simulink model "meam_simulink"  (R2020a)
settings: Solver=FixedStepAuto  StartTime=0.0  StopTime=10.0  FixedStep=0.0001  RelTol=1e-3
undefined symbols (not defined in the file): cnc_comp, ctc_switch, ctrl_at_end, ctrl_space, delta, ea_set_1, ea_set_2, ee_att_1, ee_att_2, f_des, force_ffwd, fp_1, fp_2, frc_comp, grv_comp, ip_1, ip_2, K, Kc, Kd, Kdf, Ki, Kif, Km, Kp, Kpf, orn_at_norm, prdc_frc, q_posIni, q_posIni_1, robot_model_1, robot_model_2, rpt_num_1, rpt_num_2, Sf_diag, spr_comp, switch_val, Sx_diag, tf_1, tf_2, trj_at_end, trj_profile_1, trj_profile_2, trj_space_1, trj_space_2, trj_type_1, trj_type_2
libraries: simulink x2, vrlib x1
(part 1 of 4)
settings Model: Creator=Mertcan  LastModifiedBy=Mertcan

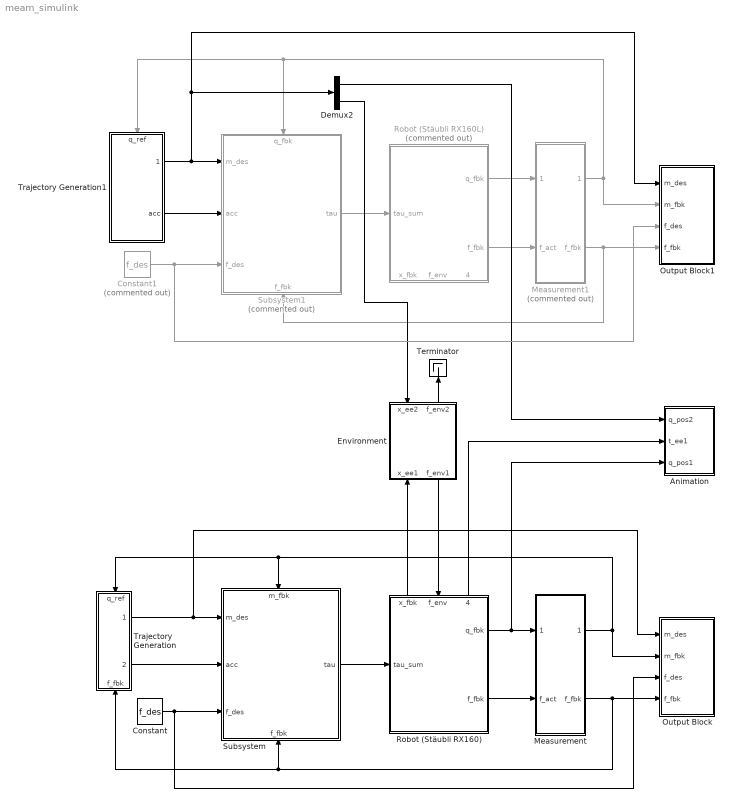
== system meam_simulink ==
  Animation : Subsystem
  Constant : Constant  Value=f_des
  Constant1 : Constant  Commented=on  Value=f_des
  Demux2 : Demux  Outputs=[12;18]
  Environment : Subsystem
      settings: PortSchema="{\"entries\":[{\"content\":{\"sides\":[{\"content\":{\"connectorIds\":[]},\"type\":\"ConnectorPlacement.EquallySpacedRectSide\",\"uuid\":\"b81f9d7c-ea51-4f8c-a6d1-c33009541a36\"},{\"content\":{\"connectorIds\":[],\"side\":\"RIGHT\"},\"type\":\"ConnectorPlacement.EquallySpacedRectSide\",\"uuid\":\"c20f2b2d-2c64-4ed8-b53c-24ad73d5cd54\"},{\"content\":{\"connectorIds\":[\"In1\",\"Out2\"],\"side\":\"TOP\"},\"type\":\"ConnectorPlacement.EquallySpacedRectSide\",\"uuid\":\"f43a164f-97c5-4b00-9b12-265fb19428de\"},{\"content\":{\"connectorIds\":[\"In2\",\"Out1\"],\"side\":\"BOTTOM\"},\"type\":\"ConnectorPlacement.EquallySpacedRectSide\",\"uuid\":\"d7f17a50-52f4-4125-8d61-9ac09671e8dc\"}]},\"type\":\"ConnectorPlacement.EquallySpacedConnector\",\"uuid\":\"950c3a05-8add-442a-8ea6-c018fdaf9f56\"}],\"packageUris\":[\"http://schema.mathworks.com/mf0/Connector/19700101\"],\"version\":\"1.0\"}"
  Measurement : Subsystem
  Measurement1 : Subsystem  Commented=on
  Output Block : Subsystem
  Output Block1 : Subsystem
  Robot (Stäubli RX160) : Subsystem
      settings: PortSchema="{\"entries\":[{\"content\":{\"sides\":[{\"content\":{\"connectorIds\":[\"In1\"]},\"type\":\"ConnectorPlacement.EquallySpacedRectSide\",\"uuid\":\"6284adc3-d758-45ef-9141-dee680c83b08\"},{\"content\":{\"connectorIds\":[\"Out1\",\"Out2\"],\"side\":\"RIGHT\"},\"type\":\"ConnectorPlacement.EquallySpacedRectSide\",\"uuid\":\"181d7ec4-49ad-445a-9254-c2b56cfcaf16\"},{\"content\":{\"connectorIds\":[\"Out3\",\"In2\",\"Out4\"],\"side\":\"TOP\"},\"type\":\"ConnectorPlacement.EquallySpacedRectSide\",\"uuid\":\"b714267f-2932-4320-9de1-3f424c8ad2a6\"}]},\"type\":\"ConnectorPlacement.EquallySpacedConnector\",\"uuid\":\"69d7b4c6-737c-4cfe-af82-254ae10a5bd4\"}],\"packageUris\":[\"http://schema.mathworks.com/mf0/Connector/19700101\"],\"version\":\"1.0\"}"
      mask Display: image('$imagefile'); % Use "Edit Image" on toolstrip to change.
  Robot (Stäubli RX160L) : Subsystem  Commented=on
      settings: PortSchema="{\"entries\":[{\"content\":{\"sides\":[{\"content\":{\"connectorIds\":[\"In1\"]},\"type\":\"ConnectorPlacement.EquallySpacedRectSide\",\"uuid\":\"6284adc3-d758-45ef-9141-dee680c83b08\"},{\"content\":{\"connectorIds\":[\"Out1\",\"Out2\"],\"side\":\"RIGHT\"},\"type\":\"ConnectorPlacement.EquallySpacedRectSide\",\"uuid\":\"181d7ec4-49ad-445a-9254-c2b56cfcaf16\"},{\"content\":{\"connectorIds\":[],\"side\":\"TOP\"},\"type\":\"ConnectorPlacement.EquallySpacedRectSide\",\"uuid\":\"b714267f-2932-4320-9de1-3f424c8ad2a6\"},{\"content\":{\"connectorIds\":[\"Out3\",\"In2\",\"Out4\"],\"side\":\"BOTTOM\"},\"type\":\"ConnectorPlacement.EquallySpacedRectSide\",\"uuid\":\"b9e977bd-f5b6-4bc7-a651-d9aa29860466\"}]},\"type\":\"ConnectorPlacement.EquallySpacedConnector\",\"uuid\":\"69d7b4c6-737c-4cfe-af82-254ae10a5bd4\"}],\"packageUris\":[\"http://schema.mathworks.com/mf0/Connector/19700101\"],\"version\":\"1.0\"}"
      mask Display: image('$imagefile'); % Use "Edit Image" on toolstrip to change.
  Subsystem : Subsystem
      settings: PortSchema="{\"entries\":[{\"content\":{\"sides\":[{\"content\":{\"connectorIds\":[\"In1\",\"In2\",\"In3\"]},\"type\":\"ConnectorPlacement.EquallySpacedRectSide\",\"uuid\":\"06a54d02-8053-40c1-91cd-d8e27b3ee47c\"},{\"content\":{\"connectorIds\":[\"Out1\"],\"side\":\"RIGHT\"},\"type\":\"ConnectorPlacement.EquallySpacedRectSide\",\"uuid\":\"4a80d155-eaa4-4553-b775-68e65830b71e\"},{\"content\":{\"connectorIds\":[\"In4\"],\"side\":\"TOP\"},\"type\":\"ConnectorPlacement.EquallySpacedRectSide\",\"uuid\":\"11a6b61a-4e29-4238-936c-c215c9d368a9\"},{\"content\":{\"connectorIds\":[\"In5\"],\"side\":\"BOTTOM\"},\"type\":\"ConnectorPlacement.EquallySpacedRectSide\",\"uuid\":\"e426367f-91c4-44b7-ba01-8266a65ceab9\"}]},\"type\":\"ConnectorPlacement.EquallySpacedConnector\",\"uuid\":\"b69ba746-893b-40a9-a2ce-44750d5af8bd\"}],\"packageUris\":[\"http://schema.mathworks.com/mf0/Connector/19700101\"],\"version\":\"1.0\"}"
  Subsystem1 : Subsystem  Commented=on
      settings: PortSchema="{\"entries\":[{\"content\":{\"sides\":[{\"content\":{\"connectorIds\":[\"In1\",\"In2\",\"In3\"]},\"type\":\"ConnectorPlacement.EquallySpacedRectSide\",\"uuid\":\"cd98d980-3223-4404-96a3-1b871aee0cda\"},{\"content\":{\"connectorIds\":[\"Out1\"],\"side\":\"RIGHT\"},\"type\":\"ConnectorPlacement.EquallySpacedRectSide\",\"uuid\":\"917be7da-8185-449c-972b-8d7b61571565\"},{\"content\":{\"connectorIds\":[\"In4\"],\"side\":\"TOP\"},\"type\":\"ConnectorPlacement.EquallySpacedRectSide\",\"uuid\":\"910fa89e-4196-4c93-9d4c-b419700893fa\"},{\"content\":{\"connectorIds\":[\"In5\"],\"side\":\"BOTTOM\"},\"type\":\"ConnectorPlacement.EquallySpacedRectSide\",\"uuid\":\"8581f1c3-c928-4a87-9392-429d43b2dbef\"}]},\"type\":\"ConnectorPlacement.EquallySpacedConnector\",\"uuid\":\"8ec3d0f0-5e55-41fc-8255-3218c3c2560b\"}],\"packageUris\":[\"http://schema.mathworks.com/mf0/Connector/19700101\"],\"version\":\"1.0\"}"
  Terminator : Terminator
  Trajectory Generation : Subsystem
      settings: PortSchema="{\"entries\":[{\"content\":{\"sides\":[{\"content\":{\"connectorIds\":[]},\"type\":\"ConnectorPlacement.EquallySpacedRectSide\",\"uuid\":\"88b86860-d81b-4a43-9b48-bb84105d3d48\"},{\"content\":{\"connectorIds\":[\"Out1\",\"Out2\"],\"side\":\"RIGHT\"},\"type\":\"ConnectorPlacement.EquallySpacedRectSide\",\"uuid\":\"c294309b-61d9-4e8b-865e-5d40c6635825\"},{\"content\":{\"connectorIds\":[\"In1\"],\"side\":\"TOP\"},\"type\":\"ConnectorPlacement.EquallySpacedRectSide\",\"uuid\":\"9b2aaf3f-7cff-4a7a-8968-0748d2e865cd\"},{\"content\":{\"connectorIds\":[\"In2\"],\"side\":\"BOTTOM\"},\"type\":\"ConnectorPlacement.EquallySpacedRectSide\",\"uuid\":\"3b326038-a616-4ec6-89ef-aa45e9a74c57\"}]},\"type\":\"ConnectorPlacement.EquallySpacedConnector\",\"uuid\":\"563f6bfd-f175-4769-9892-8fc54dd6cf01\"}],\"packageUris\":[\"http://schema.mathworks.com/mf0/Connector/19700101\"],\"version\":\"1.0\"}"
  Trajectory Generation1 : Subsystem
      settings: PortSchema="{\"entries\":[{\"content\":{\"sides\":[{\"content\":{\"connectorIds\":[]},\"type\":\"ConnectorPlacement.EquallySpacedRectSide\",\"uuid\":\"4512f7c1-141f-4ca9-8985-d7b3fc7dc203\"},{\"content\":{\"connectorIds\":[\"Out1\",\"Out2\"],\"side\":\"RIGHT\"},\"type\":\"ConnectorPlacement.EquallySpacedRectSide\",\"uuid\":\"5c5a9662-9ae9-4eb5-828e-be3fe6f4b168\"},{\"content\":{\"connectorIds\":[\"In1\"],\"side\":\"TOP\"},\"type\":\"ConnectorPlacement.EquallySpacedRectSide\",\"uuid\":\"4c26be9f-0fe4-4a1d-a76a-786ec65b737d\"},{\"content\":{\"connectorIds\":[],\"side\":\"BOTTOM\"},\"type\":\"ConnectorPlacement.EquallySpacedRectSide\",\"uuid\":\"9d756de9-72bc-4633-ac1d-40b2671d614a\"}]},\"type\":\"ConnectorPlacement.EquallySpacedConnector\",\"uuid\":\"303d3c57-cadd-4518-8f0b-ca4d9a4186ef\"}],\"packageUris\":[\"http://schema.mathworks.com/mf0/Connector/19700101\"],\"version\":\"1.0\"}"
  wires:
  Constant/1 -> Subsystem/3(f_des), Output Block/3(f_des)
  Measurement1/1(m_fbk) -> Output Block1/2(m_fbk), Trajectory Generation1/1(q_ref), Subsystem1/4(q_fbk)
  Environment/2(f_env2) -> Terminator/1
  Trajectory Generation1/1(pos&vel) -> Output Block1/1(m_des), Demux2/1, Subsystem1/1(m_des)
  Trajectory Generation/1(pos&vel) -> Output Block/1(m_des), Subsystem/1(m_des)
  Subsystem1/1(tau) -> Robot (Stäubli RX160L)/1(tau_sum)
  Robot (Stäubli RX160L)/1(q_fbk) -> Measurement1/1(q_act)
  Measurement/1(m_fbk) -> Output Block/2(m_fbk), Trajectory Generation/1(q_ref), Subsystem/4(m_fbk)
  Measurement1/2(f_fbk) -> Subsystem1/5(f_fbk), Output Block1/4(f_fbk)
  Robot (Stäubli RX160L)/2(f_fbk) -> Measurement1/2(f_act)
  Demux2/1 -> Animation/1(q_pos2)
  Subsystem/1(tau) -> Robot (Stäubli RX160)/1(tau_sum)
  Demux2/2 -> Environment/1(x_ee2)
  Environment/1(f_env1) -> Robot (Stäubli RX160)/2(f_env)
  Trajectory Generation/2(acc) -> Subsystem/2(acc)
  Robot (Stäubli RX160)/2(f_fbk) -> Measurement/2(f_act)
  Constant1/1 -> Output Block1/3(f_des), Subsystem1/3(f_des)
  Robot (Stäubli RX160)/4(x_compress) -> Animation/2(t_ee1)
  Measurement/2(f_fbk) -> Output Block/4(f_fbk), Trajectory Generation/2(f_fbk), Subsystem/5(f_fbk)
  Robot (Stäubli RX160)/1(q_fbk) -> Measurement/1(q_act), Animation/3(q_pos1)
  Robot (Stäubli RX160)/3(x_fbk) -> Environment/2(x_ee1)
  Trajectory Generation1/2(acc) -> Subsystem1/2(acc)

== system meam_simulink/Animation ==
  q_pos2 : Inport
  t_ee1 : Inport  Port=2
  q_pos1 : Inport  Port=3
  Constant : Constant  Value=1e3
  Demux : Demux  Outputs=2
  Demux1 : Demux  Outputs=2
  Demux2 : Demux  Outputs=3
  Product : Product
  Terminator{,1..3} (4 alike) : Terminator
  To Workspace1 : ToWorkspace  VariableName=eePosCompress  SaveFormat=Timeseries  SampleTime=-1
  VR Sink1 : vrlib/VR Sink  InstantiateOnLoad=on  SampleTime=0.1  ViewEnable=on  RemoteChange=off  RemoteView=off  FieldsWritten=joint_joint_1.rotation.4.1.1.double#joint_joint_2.rotation.4.1.1.double#joint_joint_3.rotation.4.1.1.double#joint_joint_4.rotation.4.1.1.double#joint_joint_5.rotation.4.1.1.double#joint_joint_6.rotation.4.1.1.double#rod_sphere.translation.3.1.1.double#joint_joint_1_0001.rotation.4.1.1.double#joint_joint_2_0001.rotation.4.1.1.double#joint_joint_3_0001.rotation.4.1.1.double#joint_joint_4_0001.rotation.4.1.1.double#joint_joint_5_0001.rotation.4.1.1.double#joint_joint_6_0001.rotation.4.1.1.double  WorldFileName=vr_two_robots_base.x3d  WorldDescription=Dual Robot Scene  AutoView=on  VideoDimensions=[]  AllowVariableSize=off  FigureProperties="{'Position', 'Name', 'Viewpoint', 'CameraBound', 'CameraDirection', 'CameraPosition', 'CameraUpVector', 'ZoomFactor', 'Antialiasing', 'Headlight', 'Lighting', 'NavPanel', 'Sound', 'StatusBar', 'Stereo3D', 'Stereo3DCameraOffset', 'Stereo3DHIT', 'ToolBar', 'Textures', 'Transparency', 'Triad', 'Wireframe', 'NavZones', 'NavMode', 'NavSpeed', 'CaptureFileFormat', 'CaptureFileName', 'Record2DCompressMethod', 'Record2DCompressQuality', 'Record2D', 'Record2DFileName', 'Record2DFPS'; [7.0100000000000000e+02   2.6000000000000000e+02   1.1860000000000000e+03   6.6700000000000000e+02], 'Dual Robot Scene', 'Close View', 'on', [9.6576292467919089e-01  -1.3282628958850401e-01   2.2284333086116798e-01], [-4.0999222072425230e+00   7.2376690346139994e-01  -4.0692759072460811e+00], [1.1281783288456564e-01   9.8854135680228927e-01   1.0029019131923340e-01], [1.0000000000000000e+00], 'on', 'on', 'on', 'halfbar', 'on', 'on', 'off', [1.0000000149011612e-01], [0.0000000000000000e+00], 'on', 'on', 'on', 'none', 'off', 'off', 'examine', 'normal', 'tif', '%f_anim_%n.tif', 'auto', [7.5000000000000000e+01], 'off', '%f_anim_%n.avi', 'auto'}"
  Zero-Order Hold : ZeroOrderHold  SampleTime=0.004
  fwd kin : MATLAB Function  TreatAsAtomicUnit=on
  fwd kin1 : MATLAB Function  TreatAsAtomicUnit=on
  wires:
  q_pos1/1 -> Demux/1
  Demux/1 -> fwd kin/1(u)
  Demux/2 -> Terminator/1
  q_pos2/1 -> Demux1/1
  Demux1/2 -> Terminator1/1
  Demux1/1 -> fwd kin1/1(u)
  fwd kin/1(r1) -> VR Sink1/1
  fwd kin/2(r2) -> VR Sink1/2
  fwd kin/3(r3) -> VR Sink1/3
  fwd kin/4(r4) -> VR Sink1/4
  fwd kin/5(r5) -> VR Sink1/5
  fwd kin/6(r6) -> VR Sink1/6
  fwd kin1/1(r1) -> VR Sink1/8
  fwd kin1/2(r2) -> VR Sink1/9
  fwd kin1/3(r3) -> VR Sink1/10
  fwd kin1/4(r4) -> VR Sink1/11
  fwd kin1/5(r5) -> VR Sink1/12
  fwd kin1/6(r6) -> VR Sink1/13
  t_ee1/1 -> Product/2, Demux2/1
  Product/1 -> VR Sink1/7
  Constant/1 -> Product/1
  Demux2/1 -> Terminator2/1
  Demux2/2 -> Terminator3/1
  Zero-Order Hold/1 -> To Workspace1/1
  Demux2/3 -> Zero-Order Hold/1

== system meam_simulink/Environment ==
  x_ee2 : Inport
  x_ee1 : Inport  Port=2
  Clock : Clock  Commented=on
  Constant : Constant  Value=-1
  Constant2 : Constant  Commented=on  Value=[0;0;0]
  MATLAB Function : MATLAB Function  Commented=on  TreatAsAtomicUnit=on
  MATLAB Function1 : MATLAB Function  TreatAsAtomicUnit=on
  MATLAB Function2 : MATLAB Function  Commented=on  TreatAsAtomicUnit=on
  MATLAB Function3 : MATLAB Function  Commented=on  TreatAsAtomicUnit=on
  Product : Product
  Scope : Scope  Commented=on
  Stifness : Constant  Commented=on  Value=K
  Stifness1 : Constant  Value=K
  To Workspace1 : ToWorkspace  Commented=on  VariableName=obsPos  SaveFormat=Timeseries  SampleTime=-1
  delta : Constant  Commented=on  Value=delta
  end-effector attach : Constant  Value=ee_att_1
  f_env1 : Outport
  f_env2 : Outport  Port=2
  wires:
  Stifness/1 -> MATLAB Function/1(K)
  Clock/1 -> MATLAB Function/4(t)
  MATLAB Function/2(x) -> To Workspace1/1, Scope/1
  delta/1 -> MATLAB Function/2(delta)
  x_ee2/1 -> MATLAB Function1/3(x2)
  Product/1 -> f_env2/1
  x_ee1/1 -> MATLAB Function1/1(x1)  "x"
  Stifness1/1 -> MATLAB Function1/4(K)
  MATLAB Function1/1(f_e) -> Product/2, f_env1/1
  Constant2/1 -> MATLAB Function/3(u)
  Constant/1 -> Product/1
  end-effector attach/1 -> MATLAB Function1/2(ee_att_1)

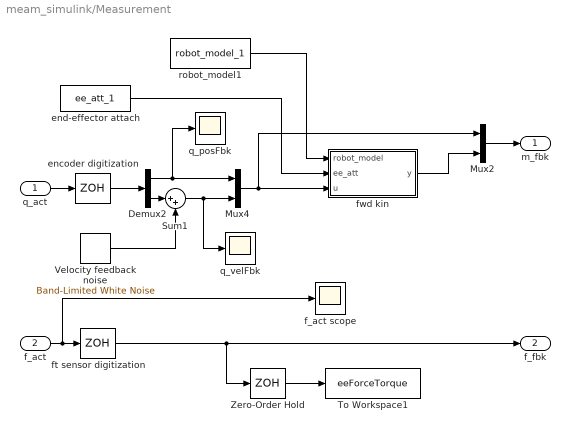
== system meam_simulink/Measurement ==
  q_act : Inport
  f_act : Inport  Port=2
  Demux2 : Demux  Outputs=2
  Mux2 : Mux  Inputs=[12;18]
  Mux4 : Mux  Inputs=2
  Sum1 : Sum  Inputs=|++
  To Workspace1 : ToWorkspace  VariableName=eeForceTorque  SaveFormat=Timeseries  SampleTime=-1
  Velocity feedback noise : simulink/Sources/Band-Limited White Noise  Cov=[0.00001]  Ts=0.01  seed=[23341]
  Zero-Order Hold : ZeroOrderHold  SampleTime=0.004
  encoder digitization : ZeroOrderHold  SampleTime=0.004
  end-effector attach : Constant  Value=ee_att_1
  f_act scope : Scope
  ft sensor digitization : ZeroOrderHold  SampleTime=0.004
  fwd kin : MATLAB Function  TreatAsAtomicUnit=on
  q_posFbk : Scope
  q_velFbk : Scope
  robot_model1 : Constant  Value=robot_model_1
  m_fbk : Outport
  f_fbk : Outport  Port=2
  wires:
  ft sensor digitization/1 -> f_fbk/1, Zero-Order Hold/1
  f_act/1 -> f_act scope/1, ft sensor digitization/1
  q_act/1 -> encoder digitization/1
  robot_model1/1 -> fwd kin/1(robot_model)
  fwd kin/1(y) -> Mux2/2
  Mux2/1 -> m_fbk/1
  Demux2/1 -> q_posFbk/1, Mux4/1
  encoder digitization/1 -> Demux2/1
  Mux4/1 -> fwd kin/3(u), Mux2/1
  Demux2/2 -> Sum1/1
  Sum1/1 -> q_velFbk/1, Mux4/2
  Velocity feedback noise/1 -> Sum1/2
  end-effector attach/1 -> fwd kin/2(ee_att)
  Zero-Order Hold/1 -> To Workspace1/1

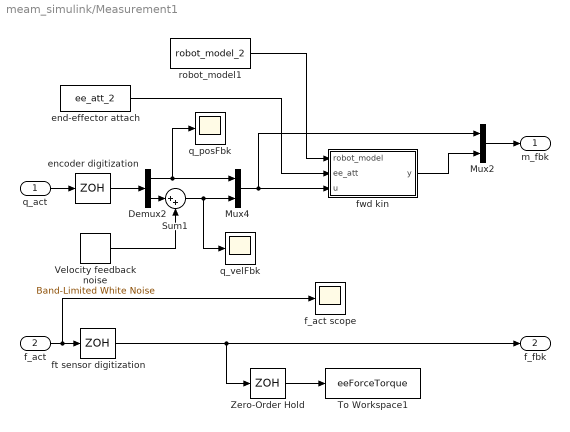
== system meam_simulink/Measurement1 ==
  q_act : Inport
  f_act : Inport  Port=2
  Demux2 : Demux  Outputs=2
  Mux2 : Mux  Inputs=[12;18]
  Mux4 : Mux  Inputs=2
  Sum1 : Sum  Inputs=|++
  To Workspace1 : ToWorkspace  VariableName=eeForceTorque  SaveFormat=Timeseries  SampleTime=-1
  Velocity feedback noise : simulink/Sources/Band-Limited White Noise  Cov=[0.00001]  Ts=0.01  seed=[23341]
  Zero-Order Hold : ZeroOrderHold  SampleTime=0.004
  encoder digitization : ZeroOrderHold  SampleTime=0.004
  end-effector attach : Constant  Value=ee_att_2
  f_act scope : Scope
  ft sensor digitization : ZeroOrderHold  SampleTime=0.004
  fwd kin : MATLAB Function  TreatAsAtomicUnit=on
  q_posFbk : Scope
  q_velFbk : Scope
  robot_model1 : Constant  Value=robot_model_2
  m_fbk : Outport
  f_fbk : Outport  Port=2
  wires:
  ft sensor digitization/1 -> f_fbk/1, Zero-Order Hold/1
  f_act/1 -> f_act scope/1, ft sensor digitization/1
  q_act/1 -> encoder digitization/1
  robot_model1/1 -> fwd kin/1(robot_model)
  fwd kin/1(y) -> Mux2/2
  Mux2/1 -> m_fbk/1
  Demux2/1 -> q_posFbk/1, Mux4/1
  encoder digitization/1 -> Demux2/1
  Mux4/1 -> fwd kin/3(u), Mux2/1
  Demux2/2 -> Sum1/1
  Sum1/1 -> q_velFbk/1, Mux4/2
  Velocity feedback noise/1 -> Sum1/2
  end-effector attach/1 -> fwd kin/2(ee_att)
  Zero-Order Hold/1 -> To Workspace1/1

== system meam_simulink/Output Block ==
  m_des : Inport
  m_fbk : Inport  Port=2
  f_des : Inport  Port=3
  f_fbk : Inport  Port=4
  Demux : Demux  Outputs=2
  Demux1 : Demux  Outputs=2
  Demux2 : Demux  Outputs=[12;18]
  Demux3 : Demux  Outputs=[12;18]
  Scope : Scope  NumInputPorts=2
  Scope1 : Scope  NumInputPorts=2
  Scope2 : Scope
  Scope3 : Scope
  Terminator{,1..3} (4 alike) : Terminator
  To Workspace : ToWorkspace  VariableName=jointPosFbk  SaveFormat=Timeseries  SampleTime=-1
  To Workspace1 : ToWorkspace  VariableName=jointPosDes  SaveFormat=Timeseries  SampleTime=-1
  wires:
  Demux/2 -> Scope1/2
  Demux1/2 -> Scope1/1
  m_des/1 -> Demux2/1
  Demux2/1 -> Demux1/1
  Demux/1 -> Scope/2, To Workspace/1
  Demux1/1 -> Scope3/1, To Workspace1/1, Scope/1
  m_fbk/1 -> Demux3/1
  Demux3/1 -> Demux/1
  Demux3/2 -> Terminator/1
  Demux2/2 -> Terminator1/1
  f_des/1 -> Terminator2/1
  f_fbk/1 -> Scope2/1, Terminator3/1

== system meam_simulink/Output Block1 ==
  m_des : Inport
  m_fbk : Inport  Port=2
  f_des : Inport  Port=3
  f_fbk : Inport  Port=4
  Demux : Demux  Commented=on  Outputs=2
  Demux1 : Demux  Outputs=2
  Demux2 : Demux  Outputs=[12;18]
  Demux3 : Demux  Commented=on  Outputs=[12;18]
  Scope : Scope  Commented=on  NumInputPorts=2
  Scope1 : Scope  Commented=on  NumInputPorts=2
  Scope2 : Scope  Commented=on
  Scope3 : Scope
  Terminator : Terminator  Commented=on
  Terminator1 : Terminator
  Terminator2 : Terminator  Commented=on
  Terminator3 : Terminator  Commented=on
  To Workspace : ToWorkspace  Commented=on  VariableName=jointPosFbk  SaveFormat=Timeseries  SampleTime=-1
  To Workspace1 : ToWorkspace  VariableName=jointPosDes2  SaveFormat=Timeseries  SampleTime=-1
  Zero-Order Hold2 : ZeroOrderHold  SampleTime=0.004
  wires:
  Demux/2 -> Scope1/2
  Demux1/2 -> Scope1/1
  m_des/1 -> Demux2/1
  Demux2/1 -> Demux1/1
  Demux/1 -> Scope/2, To Workspace/1
  Demux1/1 -> Scope3/1, Zero-Order Hold2/1, Scope/1
  m_fbk/1 -> Demux3/1
  Demux3/1 -> Demux/1
  Demux3/2 -> Terminator/1
  Demux2/2 -> Terminator1/1
  f_des/1 -> Terminator2/1
  f_fbk/1 -> Scope2/1, Terminator3/1
  Zero-Order Hold2/1 -> To Workspace1/1

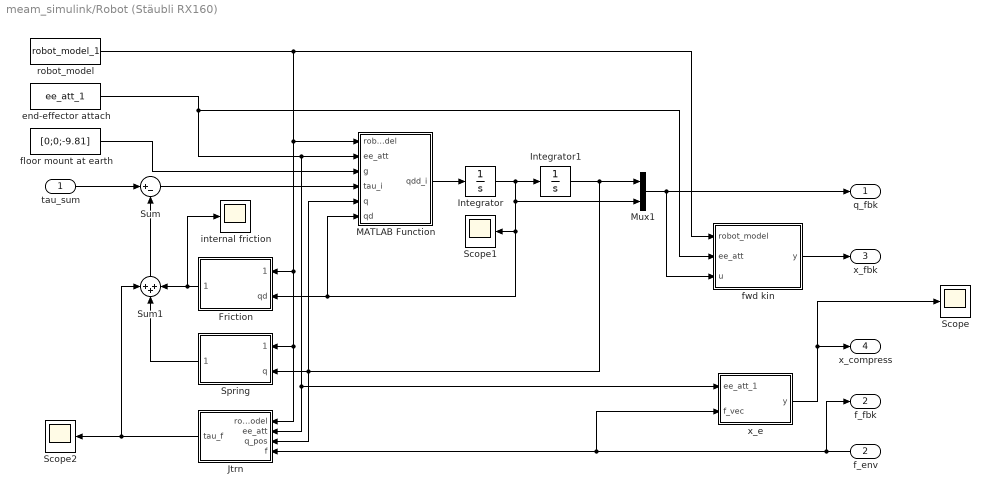
== system meam_simulink/Robot (Stäubli RX160) ==
  tau_sum : Inport
  f_env : Inport  Port=2
  Friction : MATLAB Function  TreatAsAtomicUnit=on
  Integrator : Integrator
  Integrator1 : Integrator  InitialCondition=q_posIni_1
  Jtrn : MATLAB Function  TreatAsAtomicUnit=on
  MATLAB Function : MATLAB Function  TreatAsAtomicUnit=on
  Mux1 : Mux  Inputs=2
  Scope : Scope
  Scope1 : Scope
  Scope2 : Scope
  Spring : MATLAB Function  TreatAsAtomicUnit=on
  Sum : Sum  Inputs=|+-
  Sum1 : Sum  Inputs=+++
  end-effector attach : Constant  Value=ee_att_1
  floor mount at earth : Constant  Value=[0;0;-9.81]
  fwd kin : MATLAB Function  TreatAsAtomicUnit=on
  internal friction : Scope
  robot_model : Constant  Value=robot_model_1
  x_e : MATLAB Function  TreatAsAtomicUnit=on
  q_fbk : Outport
  f_fbk : Outport  Port=2
  x_fbk : Outport  Port=3
  x_compress : Outport  Port=4
  wires:
  MATLAB Function/1(qdd_i) -> Integrator/1
  Sum/1 -> MATLAB Function/4(tau_i)
  Integrator1/1 -> Jtrn/3(q_pos), MATLAB Function/5(q), Spring/2(q), Mux1/1
  Integrator/1 -> MATLAB Function/6(qd), Friction/2(qd), Scope1/1, Mux1/2, Integrator1/1
  Friction/1(tau_frc) -> Sum1/3, internal friction/1
  Spring/1(tau_spr) -> Sum1/2
  robot_model/1 -> Jtrn/1(robot_model), Spring/1(robot_model), Friction/1(robot_model), MATLAB Function/1(robot_model), fwd kin/1(robot_model)
  Mux1/1 -> q_fbk/1, fwd kin/3(u)
  fwd kin/1(y) -> x_fbk/1
  Sum1/1 -> Sum/2
  tau_sum/1 -> Sum/1
  f_env/1 -> f_fbk/1, x_e/2(f_vec), Jtrn/4(f)
  Jtrn/1(tau_f) -> Sum1/1, Scope2/1
  end-effector attach/1 -> MATLAB Function/2(ee_att), Jtrn/2(ee_att), x_e/1(ee_att_1), fwd kin/2(ee_att)
  floor mount at earth/1 -> MATLAB Function/3(g)
  x_e/1(y) -> Scope/1, x_compress/1

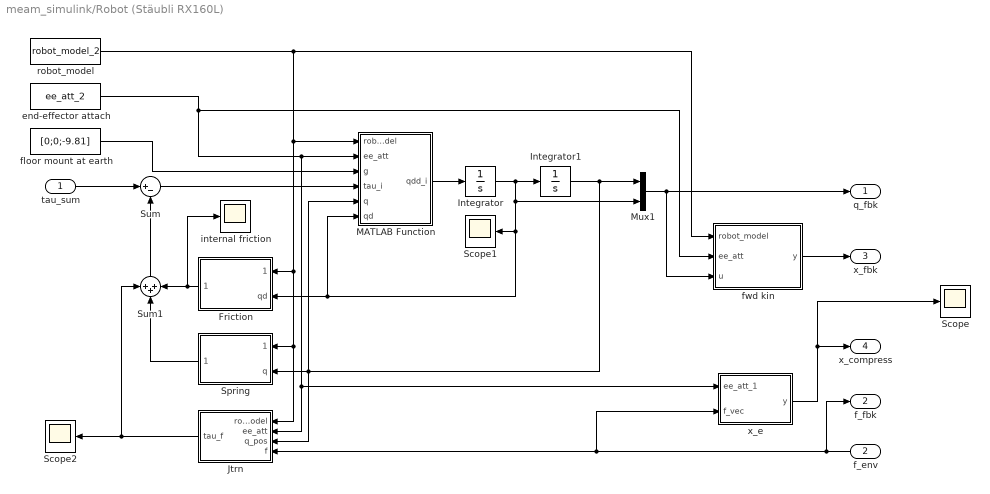
== system meam_simulink/Robot (Stäubli RX160L) ==
  tau_sum : Inport
  f_env : Inport  Port=2
  Friction : MATLAB Function  TreatAsAtomicUnit=on
  Integrator : Integrator
  Integrator1 : Integrator  InitialCondition=q_posIni
  Jtrn : MATLAB Function  TreatAsAtomicUnit=on
  MATLAB Function : MATLAB Function  TreatAsAtomicUnit=on
  Mux1 : Mux  Inputs=2
  Scope : Scope
  Scope1 : Scope
  Scope2 : Scope
  Spring : MATLAB Function  TreatAsAtomicUnit=on
  Sum : Sum  Inputs=|+-
  Sum1 : Sum  Inputs=+++
  end-effector attach : Constant  Value=ee_att_2
  floor mount at earth : Constant  Value=[0;0;-9.81]
  fwd kin : MATLAB Function  TreatAsAtomicUnit=on
  internal friction : Scope
  robot_model : Constant  Value=robot_model_2
  x_e : MATLAB Function  TreatAsAtomicUnit=on
  q_fbk : Outport
  f_fbk : Outport  Port=2
  x_fbk : Outport  Port=3
  x_compress : Outport  Port=4
  wires:
  MATLAB Function/1(qdd_i) -> Integrator/1
  Sum/1 -> MATLAB Function/4(tau_i)
  Integrator1/1 -> Jtrn/3(q_pos), MATLAB Function/5(q), Spring/2(q), Mux1/1
  Integrator/1 -> MATLAB Function/6(qd), Friction/2(qd), Scope1/1, Mux1/2, Integrator1/1
  Friction/1(tau_frc) -> Sum1/3, internal friction/1
  Spring/1(tau_spr) -> Sum1/2
  robot_model/1 -> Jtrn/1(robot_model), Spring/1(robot_model), Friction/1(robot_model), MATLAB Function/1(robot_model), fwd kin/1(robot_model)
  Mux1/1 -> q_fbk/1, fwd kin/3(u)
  fwd kin/1(y) -> x_fbk/1
  Sum1/1 -> Sum/2
  tau_sum/1 -> Sum/1
  f_env/1 -> f_fbk/1, x_e/2(f_vec), Jtrn/4(f)
  Jtrn/1(tau_f) -> Sum1/1, Scope2/1
  end-effector attach/1 -> MATLAB Function/2(ee_att), Jtrn/2(ee_att), x_e/1(ee_att_1), fwd kin/2(ee_att)
  floor mount at earth/1 -> MATLAB Function/3(g)
  x_e/1(y) -> Scope/1, x_compress/1

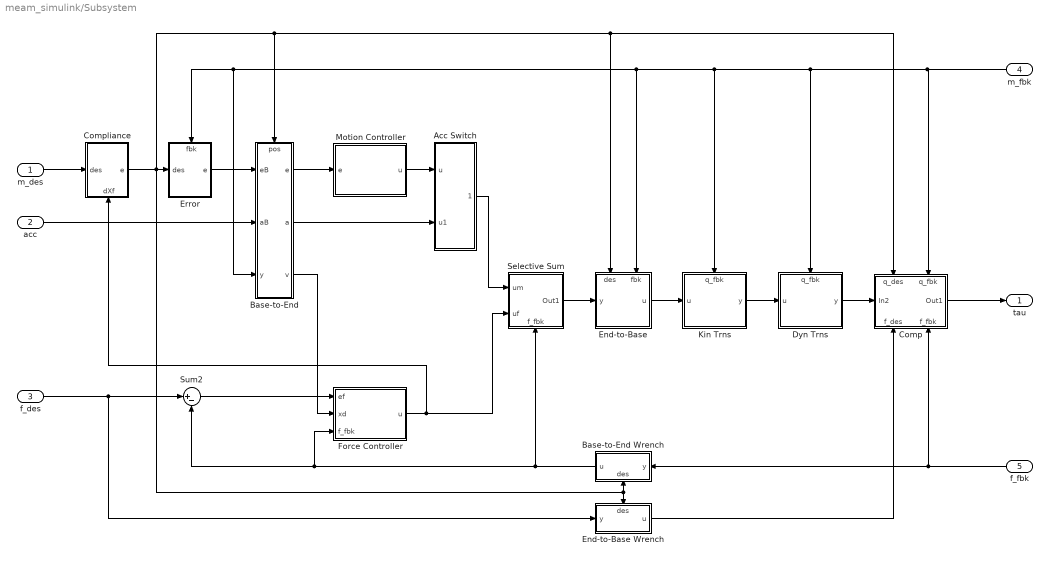
== system meam_simulink/Subsystem ==
  m_des : Inport
  acc : Inport  Port=2
  f_des : Inport  Port=3
  m_fbk : Inport  Port=4
  f_fbk : Inport  Port=5
  Acc Switch : Subsystem
  Base-to-End : Subsystem
      settings: PortSchema="{\"entries\":[{\"content\":{\"sides\":[{\"content\":{\"connectorIds\":[\"In1\",\"In2\",\"In3\"]},\"type\":\"ConnectorPlacement.EquallySpacedRectSide\",\"uuid\":\"020565b3-ffe2-42af-b350-3d5bbba08d44\"},{\"content\":{\"connectorIds\":[\"Out1\",\"Out2\",\"Out3\"],\"side\":\"RIGHT\"},\"type\":\"ConnectorPlacement.EquallySpacedRectSide\",\"uuid\":\"dbb2181b-8ce7-432e-bb43-e79a64d985e0\"},{\"content\":{\"connectorIds\":[\"In4\"],\"side\":\"TOP\"},\"type\":\"ConnectorPlacement.EquallySpacedRectSide\",\"uuid\":\"edd439a8-cf84-4371-9d31-8030538399a3\"}]},\"type\":\"ConnectorPlacement.EquallySpacedConnector\",\"uuid\":\"06f3d9c3-bbec-4c64-9009-98f920580bff\"}],\"packageUris\":[\"http://schema.mathworks.com/mf0/Connector/19700101\"],\"version\":\"1.0\"}"
  Base-to-End Wrench : Subsystem
      settings: PortSchema="{\"entries\":[{\"content\":{\"sides\":[{\"content\":{\"connectorIds\":[\"In1\"]},\"type\":\"ConnectorPlacement.EquallySpacedRectSide\",\"uuid\":\"020565b3-ffe2-42af-b350-3d5bbba08d44\"},{\"content\":{\"connectorIds\":[\"Out1\"],\"side\":\"RIGHT\"},\"type\":\"ConnectorPlacement.EquallySpacedRectSide\",\"uuid\":\"dbb2181b-8ce7-432e-bb43-e79a64d985e0\"},{\"content\":{\"connectorIds\":[],\"side\":\"TOP\"},\"type\":\"ConnectorPlacement.EquallySpacedRectSide\",\"uuid\":\"edd439a8-cf84-4371-9d31-8030538399a3\"},{\"content\":{\"connectorIds\":[\"In2\"],\"side\":\"BOTTOM\"},\"type\":\"ConnectorPlacement.EquallySpacedRectSide\",\"uuid\":\"efdc06f9-64f5-4bb4-980e-2734ab920eb4\"}]},\"type\":\"ConnectorPlacement.EquallySpacedConnector\",\"uuid\":\"06f3d9c3-bbec-4c64-9009-98f920580bff\"}],\"packageUris\":[\"http://schema.mathworks.com/mf0/Connector/19700101\"],\"version\":\"1.0\"}"
  Comp : Subsystem
      settings: PortSchema="{\"entries\":[{\"content\":{\"sides\":[{\"content\":{\"connectorIds\":[\"In1\"]},\"type\":\"ConnectorPlacement.EquallySpacedRectSide\",\"uuid\":\"b4f3562c-3a59-4f04-a3b3-da66869d7fb8\"},{\"content\":{\"connectorIds\":[\"Out1\"],\"side\":\"RIGHT\"},\"type\":\"ConnectorPlacement.EquallySpacedRectSide\",\"uuid\":\"1269bb29-09be-43cb-9af3-f74a6a005ad0\"},{\"content\":{\"connectorIds\":[\"In2\",\"In3\"],\"side\":\"TOP\"},\"type\":\"ConnectorPlacement.EquallySpacedRectSide\",\"uuid\":\"acd55610-2ecf-4dcc-b0bc-a4343bb42bde\"},{\"content\":{\"connectorIds\":[\"In4\",\"In5\"],\"side\":\"BOTTOM\"},\"type\":\"ConnectorPlacement.EquallySpacedRectSide\",\"uuid\":\"40156ef2-2d75-41dd-a033-e544f1ff9354\"}]},\"type\":\"ConnectorPlacement.EquallySpacedConnector\",\"uuid\":\"953ff7fc-1f3b-47dc-a69f-74118f573792\"}],\"packageUris\":[\"http://schema.mathworks.com/mf0/Connector/19700101\"],\"version\":\"1.0\"}"
  Compliance : Subsystem
      settings: PortSchema="{\"entries\":[{\"content\":{\"sides\":[{\"content\":{\"connectorIds\":[\"In1\"]},\"type\":\"ConnectorPlacement.EquallySpacedRectSide\",\"uuid\":\"178f6af3-2ba7-43c9-b15c-ce5e8339bdff\"},{\"content\":{\"connectorIds\":[\"Out1\"],\"side\":\"RIGHT\"},\"type\":\"ConnectorPlacement.EquallySpacedRectSide\",\"uuid\":\"a6ae646a-c86d-4621-9c36-e111e1f88696\"},{\"content\":{\"connectorIds\":[],\"side\":\"TOP\"},\"type\":\"ConnectorPlacement.EquallySpacedRectSide\",\"uuid\":\"808e2785-04c0-49cf-ade9-42ab28b9e69b\"},{\"content\":{\"connectorIds\":[\"In2\"],\"side\":\"BOTTOM\"},\"type\":\"ConnectorPlacement.EquallySpacedRectSide\",\"uuid\":\"5e5af769-b9d3-4274-a83d-533a837274af\"}]},\"type\":\"ConnectorPlacement.EquallySpacedConnector\",\"uuid\":\"8e74479a-b980-46f8-8664-436c69a1a6e0\"}],\"packageUris\":[\"http://schema.mathworks.com/mf0/Connector/19700101\"],\"version\":\"1.0\"}"
  Dyn Trns : Subsystem
      settings: PortSchema="{\"entries\":[{\"content\":{\"sides\":[{\"content\":{\"connectorIds\":[\"In1\"]},\"type\":\"ConnectorPlacement.EquallySpacedRectSide\",\"uuid\":\"b813e676-63a5-423f-a8fb-c61aa562c7ca\"},{\"content\":{\"connectorIds\":[\"Out1\"],\"side\":\"RIGHT\"},\"type\":\"ConnectorPlacement.EquallySpacedRectSide\",\"uuid\":\"4be16838-ab6b-4909-a3bd-a94cc7d57bb6\"},{\"content\":{\"connectorIds\":[\"In2\"],\"side\":\"TOP\"},\"type\":\"ConnectorPlacement.EquallySpacedRectSide\",\"uuid\":\"1ff041d7-0766-44e3-aab7-ad2a75321725\"},{\"content\":{\"connectorIds\":[],\"side\":\"BOTTOM\"},\"type\":\"ConnectorPlacement.EquallySpacedRectSide\",\"uuid\":\"f928bd91-1fe8-4da1-ba92-0943790ffd46\"}]},\"type\":\"ConnectorPlacement.EquallySpacedConnector\",\"uuid\":\"28f3288f-f4ad-4a8c-a989-5860322fd42e\"}],\"packageUris\":[\"http://schema.mathworks.com/mf0/Connector/19700101\"],\"version\":\"1.0\"}"
  End-to-Base : Subsystem
      settings: PortSchema="{\"entries\":[{\"content\":{\"sides\":[{\"content\":{\"connectorIds\":[\"In1\"]},\"type\":\"ConnectorPlacement.EquallySpacedRectSide\",\"uuid\":\"020565b3-ffe2-42af-b350-3d5bbba08d44\"},{\"content\":{\"connectorIds\":[\"Out1\"],\"side\":\"RIGHT\"},\"type\":\"ConnectorPlacement.EquallySpacedRectSide\",\"uuid\":\"dbb2181b-8ce7-432e-bb43-e79a64d985e0\"},{\"content\":{\"connectorIds\":[\"In2\",\"In3\"],\"side\":\"TOP\"},\"type\":\"ConnectorPlacement.EquallySpacedRectSide\",\"uuid\":\"edd439a8-cf84-4371-9d31-8030538399a3\"}]},\"type\":\"ConnectorPlacement.EquallySpacedConnector\",\"uuid\":\"06f3d9c3-bbec-4c64-9009-98f920580bff\"}],\"packageUris\":[\"http://schema.mathworks.com/mf0/Connector/19700101\"],\"version\":\"1.0\"}"
  End-to-Base Wrench : Subsystem
      settings: PortSchema="{\"entries\":[{\"content\":{\"sides\":[{\"content\":{\"connectorIds\":[\"In1\"]},\"type\":\"ConnectorPlacement.EquallySpacedRectSide\",\"uuid\":\"020565b3-ffe2-42af-b350-3d5bbba08d44\"},{\"content\":{\"connectorIds\":[\"Out1\"],\"side\":\"RIGHT\"},\"type\":\"ConnectorPlacement.EquallySpacedRectSide\",\"uuid\":\"dbb2181b-8ce7-432e-bb43-e79a64d985e0\"},{\"content\":{\"connectorIds\":[\"In2\"],\"side\":\"TOP\"},\"type\":\"ConnectorPlacement.EquallySpacedRectSide\",\"uuid\":\"edd439a8-cf84-4371-9d31-8030538399a3\"}]},\"type\":\"ConnectorPlacement.EquallySpacedConnector\",\"uuid\":\"06f3d9c3-bbec-4c64-9009-98f920580bff\"}],\"packageUris\":[\"http://schema.mathworks.com/mf0/Connector/19700101\"],\"version\":\"1.0\"}"
  Error : Subsystem
      settings: PortSchema="{\"entries\":[{\"content\":{\"sides\":[{\"content\":{\"connectorIds\":[\"In1\"]},\"type\":\"ConnectorPlacement.EquallySpacedRectSide\",\"uuid\":\"178f6af3-2ba7-43c9-b15c-ce5e8339bdff\"},{\"content\":{\"connectorIds\":[\"Out1\"],\"side\":\"RIGHT\"},\"type\":\"ConnectorPlacement.EquallySpacedRectSide\",\"uuid\":\"a6ae646a-c86d-4621-9c36-e111e1f88696\"},{\"content\":{\"connectorIds\":[\"In2\"],\"side\":\"TOP\"},\"type\":\"ConnectorPlacement.EquallySpacedRectSide\",\"uuid\":\"808e2785-04c0-49cf-ade9-42ab28b9e69b\"},{\"content\":{\"connectorIds\":[],\"side\":\"BOTTOM\"},\"type\":\"ConnectorPlacement.EquallySpacedRectSide\",\"uuid\":\"5e5af769-b9d3-4274-a83d-533a837274af\"}]},\"type\":\"ConnectorPlacement.EquallySpacedConnector\",\"uuid\":\"8e74479a-b980-46f8-8664-436c69a1a6e0\"}],\"packageUris\":[\"http://schema.mathworks.com/mf0/Connector/19700101\"],\"version\":\"1.0\"}"
  Force Controller : Subsystem
  Kin Trns : Subsystem
      settings: PortSchema="{\"entries\":[{\"content\":{\"sides\":[{\"content\":{\"connectorIds\":[\"In1\"]},\"type\":\"ConnectorPlacement.EquallySpacedRectSide\",\"uuid\":\"178f6af3-2ba7-43c9-b15c-ce5e8339bdff\"},{\"content\":{\"connectorIds\":[\"Out1\"],\"side\":\"RIGHT\"},\"type\":\"ConnectorPlacement.EquallySpacedRectSide\",\"uuid\":\"a6ae646a-c86d-4621-9c36-e111e1f88696\"},{\"content\":{\"connectorIds\":[\"In2\"],\"side\":\"TOP\"},\"type\":\"ConnectorPlacement.EquallySpacedRectSide\",\"uuid\":\"808e2785-04c0-49cf-ade9-42ab28b9e69b\"},{\"content\":{\"connectorIds\":[],\"side\":\"BOTTOM\"},\"type\":\"ConnectorPlacement.EquallySpacedRectSide\",\"uuid\":\"859c665c-c9df-42d0-801f-28168852978e\"}]},\"type\":\"ConnectorPlacement.EquallySpacedConnector\",\"uuid\":\"8e74479a-b980-46f8-8664-436c69a1a6e0\"}],\"packageUris\":[\"http://schema.mathworks.com/mf0/Connector/19700101\"],\"version\":\"1.0\"}"
  Motion Controller : Subsystem
  Selective Sum : Subsystem
      settings: PortSchema="{\"entries\":[{\"content\":{\"sides\":[{\"content\":{\"connectorIds\":[\"In1\",\"In2\"]},\"type\":\"ConnectorPlacement.EquallySpacedRectSide\",\"uuid\":\"dbbbc107-fbc8-47f5-9d95-7600de16627b\"},{\"content\":{\"connectorIds\":[\"Out1\"],\"side\":\"RIGHT\"},\"type\":\"ConnectorPlacement.EquallySpacedRectSide\",\"uuid\":\"8787e853-c330-4d61-8f58-c17085830519\"},{\"content\":{\"connectorIds\":[],\"side\":\"TOP\"},\"type\":\"ConnectorPlacement.EquallySpacedRectSide\",\"uuid\":\"f03d7db1-6e8a-4daf-a27a-f65505c3a089\"},{\"content\":{\"connectorIds\":[\"In3\"],\"side\":\"BOTTOM\"},\"type\":\"ConnectorPlacement.EquallySpacedRectSide\",\"uuid\":\"fa988798-1e34-4fa1-8ebc-2815db113161\"}]},\"type\":\"ConnectorPlacement.EquallySpacedConnector\",\"uuid\":\"12668bfd-1d91-401f-8203-13ab9cac1f2c\"}],\"packageUris\":[\"http://schema.mathworks.com/mf0/Connector/19700101\"],\"version\":\"1.0\"}"
  Sum2 : Sum  Inputs=|+-
  tau : Outport
  wires:
  End-to-Base/1(u) -> Kin Trns/1(u)
  Dyn Trns/1(y) -> Comp/1(In2)
  Compliance/1(e) -> End-to-Base Wrench/2(des), Base-to-End Wrench/2(des), Comp/2(q_des), End-to-Base/2(des), Base-to-End/4(pos), Error/1(des)
  Force Controller/1(u) -> Compliance/2(dXf), Selective Sum/2(uf)
  Base-to-End/3(v) -> Force Controller/2(xd)
  f_des/1 -> Sum2/1, End-to-Base Wrench/1(y)
  Base-to-End/1(e) -> Motion Controller/1(e)
  Acc Switch/1(Out1) -> Selective Sum/1(um)
  Sum2/1 -> Force Controller/1(ef)
  f_fbk/1 -> Comp/5(f_fbk), Base-to-End Wrench/1(y)
  Error/1(e) -> Base-to-End/1(eB)
  Comp/1(Out1) -> tau/1
  Base-to-End Wrench/1(u) -> Selective Sum/3(f_fbk), Force Controller/3(f_fbk), Sum2/2
  Kin Trns/1(y) -> Dyn Trns/1(u)
  Base-to-End/2(a) -> Acc Switch/2(u1)
  Selective Sum/1(Out1) -> End-to-Base/1(y)
  End-to-Base Wrench/1(u) -> Comp/4(f_des)
  Motion Controller/1(u) -> Acc Switch/1(u)
  m_des/1 -> Compliance/1(des)
  acc/1 -> Base-to-End/2(aB)
  m_fbk/1 -> Comp/3(q_fbk), Dyn Trns/2(q_fbk), Kin Trns/2(q_fbk), End-to-Base/3(fbk), Base-to-End/3(y), Error/2(fbk)

== system meam_simulink/Subsystem1 ==
  m_des : Inport
  acc : Inport  Port=2
  f_des : Inport  Port=3
  q_fbk : Inport  Port=4
  f_fbk : Inport  Port=5
  Acc Switch : Subsystem  Commented=on
  Comp : Subsystem  Commented=on
      settings: PortSchema="{\"entries\":[{\"content\":{\"sides\":[{\"content\":{\"connectorIds\":[\"In1\"]},\"type\":\"ConnectorPlacement.EquallySpacedRectSide\",\"uuid\":\"b4f3562c-3a59-4f04-a3b3-da66869d7fb8\"},{\"content\":{\"connectorIds\":[\"Out1\"],\"side\":\"RIGHT\"},\"type\":\"ConnectorPlacement.EquallySpacedRectSide\",\"uuid\":\"1269bb29-09be-43cb-9af3-f74a6a005ad0\"},{\"content\":{\"connectorIds\":[\"In2\",\"In3\"],\"side\":\"TOP\"},\"type\":\"ConnectorPlacement.EquallySpacedRectSide\",\"uuid\":\"acd55610-2ecf-4dcc-b0bc-a4343bb42bde\"},{\"content\":{\"connectorIds\":[\"In4\",\"In5\"],\"side\":\"BOTTOM\"},\"type\":\"ConnectorPlacement.EquallySpacedRectSide\",\"uuid\":\"40156ef2-2d75-41dd-a033-e544f1ff9354\"}]},\"type\":\"ConnectorPlacement.EquallySpacedConnector\",\"uuid\":\"953ff7fc-1f3b-47dc-a69f-74118f573792\"}],\"packageUris\":[\"http://schema.mathworks.com/mf0/Connector/19700101\"],\"version\":\"1.0\"}"
  Dyn Trns : Subsystem  Commented=on
      settings: PortSchema="{\"entries\":[{\"content\":{\"sides\":[{\"content\":{\"connectorIds\":[\"In1\"]},\"type\":\"ConnectorPlacement.EquallySpacedRectSide\",\"uuid\":\"b813e676-63a5-423f-a8fb-c61aa562c7ca\"},{\"content\":{\"connectorIds\":[\"Out1\"],\"side\":\"RIGHT\"},\"type\":\"ConnectorPlacement.EquallySpacedRectSide\",\"uuid\":\"4be16838-ab6b-4909-a3bd-a94cc7d57bb6\"},{\"content\":{\"connectorIds\":[\"In2\"],\"side\":\"TOP\"},\"type\":\"ConnectorPlacement.EquallySpacedRectSide\",\"uuid\":\"1ff041d7-0766-44e3-aab7-ad2a75321725\"},{\"content\":{\"connectorIds\":[],\"side\":\"BOTTOM\"},\"type\":\"ConnectorPlacement.EquallySpacedRectSide\",\"uuid\":\"f928bd91-1fe8-4da1-ba92-0943790ffd46\"}]},\"type\":\"ConnectorPlacement.EquallySpacedConnector\",\"uuid\":\"28f3288f-f4ad-4a8c-a989-5860322fd42e\"}],\"packageUris\":[\"http://schema.mathworks.com/mf0/Connector/19700101\"],\"version\":\"1.0\"}"
  Error : Subsystem  Commented=on
      settings: PortSchema="{\"entries\":[{\"content\":{\"sides\":[{\"content\":{\"connectorIds\":[\"In1\"]},\"type\":\"ConnectorPlacement.EquallySpacedRectSide\",\"uuid\":\"178f6af3-2ba7-43c9-b15c-ce5e8339bdff\"},{\"content\":{\"connectorIds\":[\"Out1\"],\"side\":\"RIGHT\"},\"type\":\"ConnectorPlacement.EquallySpacedRectSide\",\"uuid\":\"a6ae646a-c86d-4621-9c36-e111e1f88696\"},{\"content\":{\"connectorIds\":[\"In2\"],\"side\":\"TOP\"},\"type\":\"ConnectorPlacement.EquallySpacedRectSide\",\"uuid\":\"808e2785-04c0-49cf-ade9-42ab28b9e69b\"},{\"content\":{\"connectorIds\":[],\"side\":\"BOTTOM\"},\"type\":\"ConnectorPlacement.EquallySpacedRectSide\",\"uuid\":\"5e5af769-b9d3-4274-a83d-533a837274af\"}]},\"type\":\"ConnectorPlacement.EquallySpacedConnector\",\"uuid\":\"8e74479a-b980-46f8-8664-436c69a1a6e0\"}],\"packageUris\":[\"http://schema.mathworks.com/mf0/Connector/19700101\"],\"version\":\"1.0\"}"
  Force Controller : Subsystem  Commented=on
  Kin Trns : Subsystem  Commented=on
      settings: PortSchema="{\"entries\":[{\"content\":{\"sides\":[{\"content\":{\"connectorIds\":[\"In1\"]},\"type\":\"ConnectorPlacement.EquallySpacedRectSide\",\"uuid\":\"178f6af3-2ba7-43c9-b15c-ce5e8339bdff\"},{\"content\":{\"connectorIds\":[\"Out1\"],\"side\":\"RIGHT\"},\"type\":\"ConnectorPlacement.EquallySpacedRectSide\",\"uuid\":\"a6ae646a-c86d-4621-9c36-e111e1f88696\"},{\"content\":{\"connectorIds\":[\"In2\"],\"side\":\"TOP\"},\"type\":\"ConnectorPlacement.EquallySpacedRectSide\",\"uuid\":\"808e2785-04c0-49cf-ade9-42ab28b9e69b\"},{\"content\":{\"connectorIds\":[],\"side\":\"BOTTOM\"},\"type\":\"ConnectorPlacement.EquallySpacedRectSide\",\"uuid\":\"859c665c-c9df-42d0-801f-28168852978e\"}]},\"type\":\"ConnectorPlacement.EquallySpacedConnector\",\"uuid\":\"8e74479a-b980-46f8-8664-436c69a1a6e0\"}],\"packageUris\":[\"http://schema.mathworks.com/mf0/Connector/19700101\"],\"version\":\"1.0\"}"
  Motion Controller : Subsystem  Commented=on
  Scope : Scope
  Selective Sum : Subsystem  Commented=on
      settings: PortSchema="{\"entries\":[{\"content\":{\"sides\":[{\"content\":{\"connectorIds\":[\"In1\",\"In2\"]},\"type\":\"ConnectorPlacement.EquallySpacedRectSide\",\"uuid\":\"dbbbc107-fbc8-47f5-9d95-7600de16627b\"},{\"content\":{\"connectorIds\":[\"Out1\"],\"side\":\"RIGHT\"},\"type\":\"ConnectorPlacement.EquallySpacedRectSide\",\"uuid\":\"8787e853-c330-4d61-8f58-c17085830519\"},{\"content\":{\"connectorIds\":[],\"side\":\"TOP\"},\"type\":\"ConnectorPlacement.EquallySpacedRectSide\",\"uuid\":\"f03d7db1-6e8a-4daf-a27a-f65505c3a089\"},{\"content\":{\"connectorIds\":[\"In3\"],\"side\":\"BOTTOM\"},\"type\":\"ConnectorPlacement.EquallySpacedRectSide\",\"uuid\":\"fa988798-1e34-4fa1-8ebc-2815db113161\"}]},\"type\":\"ConnectorPlacement.EquallySpacedConnector\",\"uuid\":\"12668bfd-1d91-401f-8203-13ab9cac1f2c\"}],\"packageUris\":[\"http://schema.mathworks.com/mf0/Connector/19700101\"],\"version\":\"1.0\"}"
  Sum2 : Sum  Commented=on  Inputs=|+-
  tau : Outport
  wires:
  Force Controller/1(u) -> Selective Sum/2(uf)
  Motion Controller/1(u) -> Acc Switch/1(In1)
  Comp/1(Out1) -> tau/1
  Acc Switch/1(Out1) -> Selective Sum/1(um)
  Error/1(e) -> Motion Controller/1(e)
  Kin Trns/1(y) -> Dyn Trns/1(u)
  f_fbk/1 -> Comp/5(f_fbk), Selective Sum/3(f_fbk), Sum2/2
  Selective Sum/1(Out1) -> Kin Trns/1(u)
  q_fbk/1 -> Error/2(fbk), Force Controller/2(xd), Kin Trns/2(q_fbk), Dyn Trns/2(q_fbk), Comp/3(q_fbk)
  Sum2/1 -> Force Controller/1(ef)
  Dyn Trns/1(y) -> Comp/1(In2)
  m_des/1 -> Scope/1, Comp/2(q_des), Error/1(des)
  acc/1 -> Acc Switch/2(In2)
  f_des/1 -> Comp/4(f_des), Sum2/1

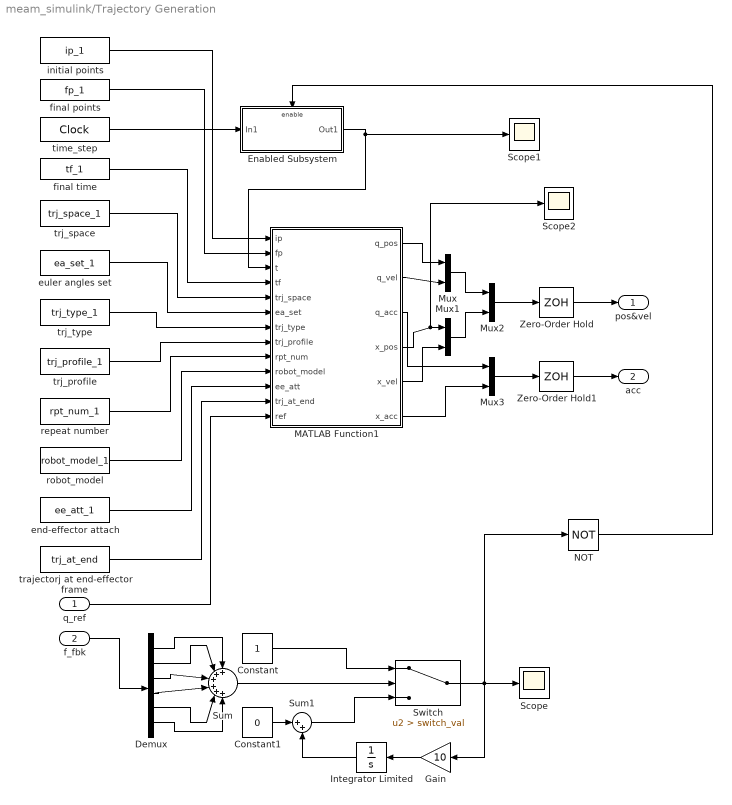
== system meam_simulink/Trajectory Generation ==
  q_ref : Inport
  f_fbk : Inport  Port=2
  Constant : Constant
  Constant1 : Constant  Value=0
  Demux : Demux  Outputs=6
  Enabled Subsystem : Subsystem  TreatAsAtomicUnit=on
  Gain : Gain  Gain=10
  Integrator Limited : Integrator  LimitOutput=on  UpperSaturationLimit=1  LowerSaturationLimit=0
  MATLAB Function1 : MATLAB Function  TreatAsAtomicUnit=on
  Mux{,1..3} (4 alike) : Mux  Inputs=2
  NOT : Logic  Operator=NOT  IconShape=distinctive  AllPortsSameDT=off  OutDataTypeStr=boolean
  Scope : Scope
  Scope1 : Scope
  Scope2 : Scope
  Sum : Sum  Inputs=++++++
  Sum1 : Sum  Inputs=|++
  Switch : Switch  Criteria=u2 > Threshold  Threshold=switch_val
  Zero-Order Hold : ZeroOrderHold  SampleTime=0.004
  Zero-Order Hold1 : ZeroOrderHold  SampleTime=0.004
  end-effector attach : Constant  Value=ee_att_1
  euler angles set : Constant  Value=ea_set_1
  final points : Constant  Value=fp_1
  final time : Constant  Value=tf_1
  initial points : Constant  Value=ip_1
  repeat number : Constant  Value=rpt_num_1
  robot_model : Constant  Value=robot_model_1
  time_step : DigitalClock  SampleTime=0.004
  trajectorj at end-effector frame : Constant  Value=trj_at_end
  trj_profile : Constant  Value=trj_profile_1
  trj_space : Constant  Value=trj_space_1
  trj_type : Constant  Value=trj_type_1
  pos&vel : Outport
  acc : Outport  Port=2
  wires:
  trj_profile/1 -> MATLAB Function1/8(trj_profile)
  MATLAB Function1/1(q_pos) -> Mux/1
  robot_model/1 -> MATLAB Function1/10(robot_model)
  initial points/1 -> MATLAB Function1/1(ip)
  final time/1 -> MATLAB Function1/4(tf)
  final points/1 -> MATLAB Function1/2(fp)
  MATLAB Function1/2(q_vel) -> Mux/2
  trj_space/1 -> MATLAB Function1/5(trj_space)
  MATLAB Function1/5(x_vel) -> Mux1/2
  MATLAB Function1/4(x_pos) -> Scope2/1, Mux1/1
  Mux2/1 -> Zero-Order Hold/1
  Mux1/1 -> Mux2/2
  Mux/1 -> Mux2/1
  q_ref/1 -> MATLAB Function1/13(ref)
  Zero-Order Hold/1 -> pos&vel/1
  MATLAB Function1/3(q_acc) -> Mux3/1
  MATLAB Function1/6(x_acc) -> Mux3/2
  Mux3/1 -> Zero-Order Hold1/1
  euler angles set/1 -> MATLAB Function1/6(ea_set)
  Zero-Order Hold1/1 -> acc/1
  trj_type/1 -> MATLAB Function1/7(trj_type)
  end-effector attach/1 -> MATLAB Function1/11(ee_att)
  repeat number/1 -> MATLAB Function1/9(rpt_num)
  trajectorj at end-effector frame/1 -> MATLAB Function1/12(trj_at_end)
  f_fbk/1 -> Demux/1
  Demux/1 -> Sum/1
  Demux/2 -> Sum/2
  Demux/3 -> Sum/3
  Demux/4 -> Sum/4
  Demux/5 -> Sum/5
  Demux/6 -> Sum/6
  Sum/1 -> Switch/2
  Constant/1 -> Switch/1
  Sum1/1 -> Switch/3
  Switch/1 -> Scope/1, NOT/1, Gain/1
  Constant1/1 -> Sum1/1
  Integrator Limited/1 -> Sum1/2
  Gain/1 -> Integrator Limited/1
  time_step/1 -> Enabled Subsystem/1(In1)
  Enabled Subsystem/1(Out1) -> Scope1/1, MATLAB Function1/3(t)
  NOT/1 -> Enabled Subsystem/Enable

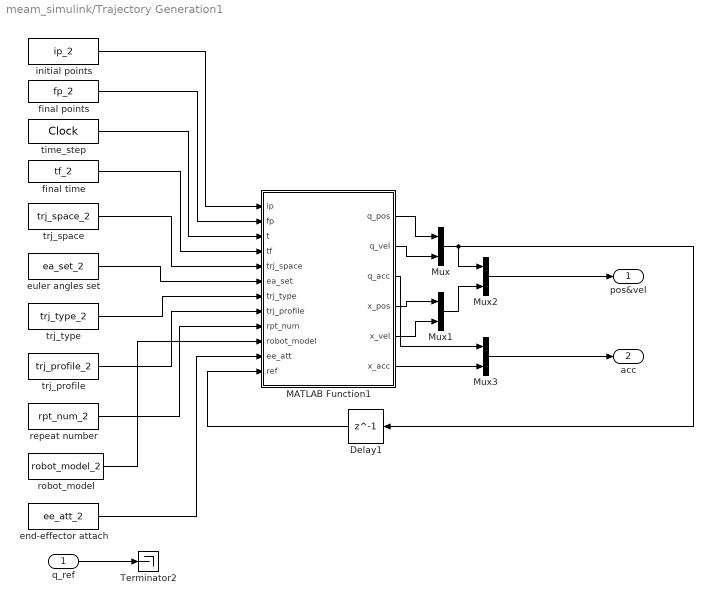
== system meam_simulink/Trajectory Generation1 ==
  q_ref : Inport
  Delay1 : Delay  DelayLength=1  InitialCondition=0
  MATLAB Function1 : MATLAB Function  TreatAsAtomicUnit=on
  Mux{,1..3} (4 alike) : Mux  Inputs=2
  Terminator2 : Terminator
  end-effector attach : Constant  Value=ee_att_2
  euler angles set : Constant  Value=ea_set_2
  final points : Constant  Value=fp_2
  final time : Constant  Value=tf_2
  initial points : Constant  Value=ip_2
  repeat number : Constant  Value=rpt_num_2
  robot_model : Constant  Value=robot_model_2
  time_step : DigitalClock  SampleTime=0.004
  trj_profile : Constant  Value=trj_profile_2
  trj_space : Constant  Value=trj_space_2
  trj_type : Constant  Value=trj_type_2
  pos&vel : Outport
  acc : Outport  Port=2
  wires:
  trj_profile/1 -> MATLAB Function1/8(trj_profile)
  time_step/1 -> MATLAB Function1/3(t)
  robot_model/1 -> MATLAB Function1/10(robot_model)
  initial points/1 -> MATLAB Function1/1(ip)
  final time/1 -> MATLAB Function1/4(tf)
  final points/1 -> MATLAB Function1/2(fp)
  MATLAB Function1/2(q_vel) -> Mux/2
  trj_space/1 -> MATLAB Function1/5(trj_space)
  MATLAB Function1/5(x_vel) -> Mux1/2
  MATLAB Function1/4(x_pos) -> Mux1/1
  Mux1/1 -> Mux2/2
  Mux2/1 -> pos&vel/1
  MATLAB Function1/3(q_acc) -> Mux3/1
  MATLAB Function1/6(x_acc) -> Mux3/2
  euler angles set/1 -> MATLAB Function1/6(ea_set)
  Mux3/1 -> acc/1
  trj_type/1 -> MATLAB Function1/7(trj_type)
  end-effector attach/1 -> MATLAB Function1/11(ee_att)
  repeat number/1 -> MATLAB Function1/9(rpt_num)
  MATLAB Function1/1(q_pos) -> Mux/1
  q_ref/1 -> Terminator2/1
  Delay1/1 -> MATLAB Function1/12(ref)
  Mux/1 -> Mux2/1, Delay1/1

== system meam_simulink/Subsystem/Acc Switch ==
  u : Inport  PortDimensions=6
  u1 : Inport  Port=2  PortDimensions=6
  Sum : Sum  Inputs=++|
  Switch : Switch  Criteria=u2 > Threshold
  computed torque switch : Constant  Value=ctc_switch
  Out1 : Outport  PortDimensions=6
  wires:
  Sum/1 -> Switch/1
  computed torque switch/1 -> Switch/2
  Switch/1 -> Out1/1
  u/1 -> Switch/3, Sum/1
  u1/1 -> Sum/2

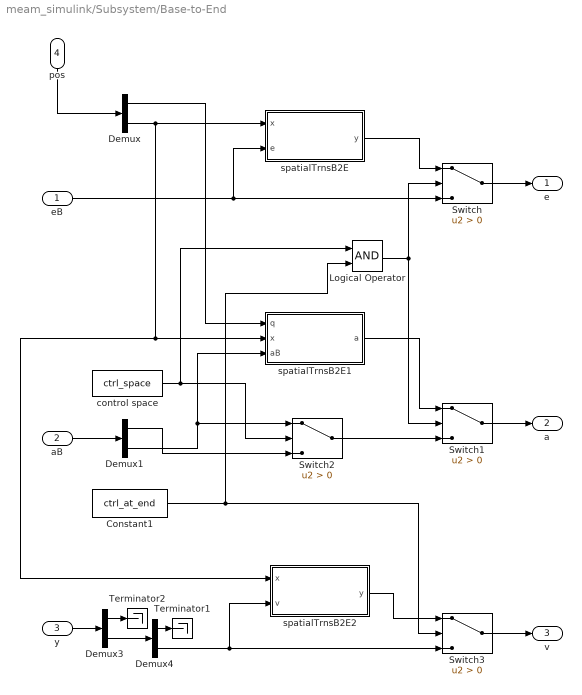
== system meam_simulink/Subsystem/Base-to-End ==
  eB : Inport  PortDimensions=12
  aB : Inport  Port=2  PortDimensions=12
  y : Inport  Port=3  PortDimensions=30
  pos : Inport  Port=4  PortDimensions=30
  Constant1 : Constant  Value=ctrl_at_end
  Demux : Demux  Outputs=[12;18]
  Demux1 : Demux  Outputs=2
  Demux3 : Demux  Outputs=[12;18]
  Demux4 : Demux  Outputs=[12;6]
  Logical Operator : Logic  AllPortsSameDT=off  OutDataTypeStr=boolean
  Switch{,1..3} (4 alike) : Switch  Criteria=u2 > Threshold
  Terminator1 : Terminator
  Terminator2 : Terminator
  control space : Constant  Value=ctrl_space
  spatialTrnsB2E : MATLAB Function  TreatAsAtomicUnit=on
  spatialTrnsB2E1 : MATLAB Function  TreatAsAtomicUnit=on
  spatialTrnsB2E2 : MATLAB Function  TreatAsAtomicUnit=on
  e : Outport  PortDimensions=12
  a : Outport  Port=2  PortDimensions=6
  v : Outport  Port=3  PortDimensions=6
  wires:
  spatialTrnsB2E/1(y) -> Switch/1
  Demux/1 -> spatialTrnsB2E1/1(q)
  pos/1 -> Demux/1
  eB/1 -> Switch/3, spatialTrnsB2E/2(e)
  Switch/1 -> e/1
  Switch1/1 -> a/1
  spatialTrnsB2E1/1(a) -> Switch1/1
  Logical Operator/1 -> Switch1/2, Switch/2
  control space/1 -> Logical Operator/1, Switch2/2
  aB/1 -> Demux1/1
  Demux1/2 -> Switch2/1, spatialTrnsB2E1/3(aB)
  Switch2/1 -> Switch1/3
  Demux1/1 -> Switch2/3
  Demux3/1 -> Terminator2/1
  y/1 -> Demux3/1
  Demux/2 -> spatialTrnsB2E1/2(x), spatialTrnsB2E2/1(x), spatialTrnsB2E/1(x)
  Demux4/1 -> Terminator1/1
  Demux3/2 -> Demux4/1
  Switch3/1 -> v/1
  spatialTrnsB2E2/1(y) -> Switch3/1
  Demux4/2 -> spatialTrnsB2E2/2(v), Switch3/3
  Constant1/1 -> Logical Operator/2, Switch3/2

== system meam_simulink/Subsystem/Base-to-End Wrench ==
  y : Inport  PortDimensions=6
  des : Inport  Port=2  PortDimensions=30
  Constant2 : Constant  Value=ctrl_at_end
  Demux : Demux  Outputs=[12;18]
  Switch : Switch  Criteria=u2 > Threshold
  Terminator : Terminator
  f_fbk scope : Scope
  spatialTrnsB2E : MATLAB Function  TreatAsAtomicUnit=on
  u : Outport  PortDimensions=6
  wires:
  y/1 -> Switch/3, spatialTrnsB2E/2(f_fbk)
  spatialTrnsB2E/1(f_fbkE) -> Switch/1
  Constant2/1 -> Switch/2
  des/1 -> Demux/1
  Demux/2 -> spatialTrnsB2E/1(x)
  Demux/1 -> Terminator/1
  Switch/1 -> f_fbk scope/1, u/1

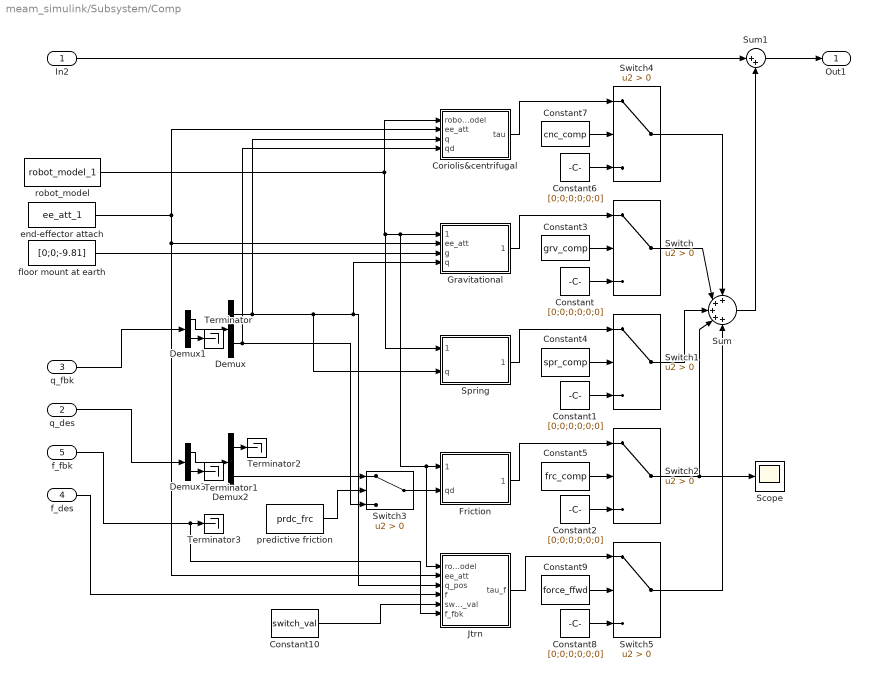
== system meam_simulink/Subsystem/Comp ==
  In2 : Inport  PortDimensions=6
  q_des : Inport  Port=2  PortDimensions=30
  q_fbk : Inport  Port=3  PortDimensions=30
  f_des : Inport  Port=4  PortDimensions=6
  f_fbk : Inport  Port=5  PortDimensions=6
  Constant{,1..2,6,8} (5 alike) : Constant  Value=[0;0;0;0;0;0]
  Constant10 : Constant  Value=switch_val
  Constant3 : Constant  Value=grv_comp
  Constant4 : Constant  Value=spr_comp
  Constant5 : Constant  Value=frc_comp
  Constant7 : Constant  Value=cnc_comp
  Constant9 : Constant  Value=force_ffwd
  Coriolis&centrifugal : MATLAB Function  TreatAsAtomicUnit=on
  Demux : Demux  Outputs=2
  Demux1 : Demux  Outputs=[12;18]
  Demux2 : Demux  Outputs=2
  Demux3 : Demux  Outputs=[12;18]
  Friction : MATLAB Function  TreatAsAtomicUnit=on
  Gravitational : MATLAB Function  TreatAsAtomicUnit=on
  Jtrn : MATLAB Function  TreatAsAtomicUnit=on
  Scope : Scope
  Spring : MATLAB Function  TreatAsAtomicUnit=on
  Sum : Sum  Inputs=+++++
  Sum1 : Sum  Inputs=|++
  Switch{,1..5} (6 alike) : Switch  Criteria=u2 > Threshold
  Terminator{,1..3} (4 alike) : Terminator
  end-effector attach : Constant  Value=ee_att_1
  floor mount at earth : Constant  Value=[0;0;-9.81]
  predictive friction : Constant  Value=prdc_frc
  robot_model : Constant  Value=robot_model_1
  Out1 : Outport  PortDimensions=6
  wires:
  Sum/1 -> Sum1/2
  Sum1/1 -> Out1/1
  In2/1 -> Sum1/1
  Constant7/1 -> Switch4/2
  Switch1/1 -> Sum/3
  Coriolis&centrifugal/1(tau) -> Switch4/1
  Switch4/1 -> Sum/1
  Demux2/2 -> Switch3/1
  f_fbk/1 -> Jtrn/6(f_fbk), Terminator3/1
  Constant6/1 -> Switch4/3
  q_des/1 -> Demux3/1
  Demux2/1 -> Terminator2/1
  Constant/1 -> Switch/3
  Demux3/2 -> Terminator1/1
  Demux1/1 -> Demux/1
  Constant5/1 -> Switch2/2
  predictive friction/1 -> Switch3/2
  Constant4/1 -> Switch1/2
  Switch/1 -> Sum/2
  robot_model/1 -> Coriolis&centrifugal/1(robot_model), Jtrn/1(robot_model), Friction/1(robot_model), Gravitational/1(robot_model), Spring/1(robot_model)
  q_fbk/1 -> Demux1/1
  Demux3/1 -> Demux2/1
  Spring/1(tau_spr) -> Switch1/1
  Switch2/1 -> Scope/1, Sum/4
  Constant1/1 -> Switch1/3
  Demux/1 -> Jtrn/3(q_pos), Gravitational/4(q), Spring/2(q), Coriolis&centrifugal/3(q)
  Friction/1(tau_frc) -> Switch2/1
  Gravitational/1(tau_grv) -> Switch/1
  Demux1/2 -> Terminator/1
  Demux/2 -> Coriolis&centrifugal/4(qd), Switch3/3
  Constant3/1 -> Switch/2
  Constant2/1 -> Switch2/3
  Switch3/1 -> Friction/2(qd)
  Constant8/1 -> Switch5/3
  Constant9/1 -> Switch5/2
  Jtrn/1(tau_f) -> Switch5/1
  Switch5/1 -> Sum/5
  floor mount at earth/1 -> Gravitational/3(g)
  end-effector attach/1 -> Jtrn/2(ee_att), Gravitational/2(ee_att), Coriolis&centrifugal/2(ee_att)
  f_des/1 -> Jtrn/4(f)
  Constant10/1 -> Jtrn/5(switch_val)

== system meam_simulink/Subsystem/Compliance ==
  des : Inport  PortDimensions=30
  dXf : Inport  Port=2  PortDimensions=6
  Compliance gain : Constant  Value=Kc
  Integrator : Integrator
  MATLAB Function : MATLAB Function  TreatAsAtomicUnit=on
  Subsystem : Subsystem  Commented=on
  Switch : Switch  Criteria=u2 > Threshold
  Zero-Order Hold : ZeroOrderHold  SampleTime=0.004
  control_space : Constant  Value=orn_at_norm
  e : Outport  PortDimensions=30
  wires:
  control_space/1 -> Switch/2
  MATLAB Function/1(y) -> Zero-Order Hold/1
  Switch/1 -> e/1
  des/1 -> Switch/3, MATLAB Function/1(des)
  dXf/1 -> Integrator/1
  Zero-Order Hold/1 -> Switch/1
  Compliance gain/1 -> MATLAB Function/2(Kc)
  Integrator/1 -> MATLAB Function/3(dXf)

== system meam_simulink/Subsystem/Dyn Trns ==
  u : Inport
  q_fbk : Inport  Port=2
  Demux : Demux  Outputs=[6;6]
  Demux1 : Demux  Outputs=[12;18]
  MATLAB Function : MATLAB Function  TreatAsAtomicUnit=on
  Switch : Switch  Criteria=u2 > Threshold
  Terminator : Terminator
  Terminator1 : Terminator
  computed torque switch : Constant  Value=ctc_switch
  end-effector attach : Constant  Value=ee_att_1
  robot_model : Constant  Value=robot_model_1
  y : Outport
  wires:
  u/1 -> Switch/3, MATLAB Function/3(u)
  robot_model/1 -> MATLAB Function/1(robot_model)
  q_fbk/1 -> Demux1/1
  Demux/1 -> MATLAB Function/4(q)
  Demux1/1 -> Demux/1
  Demux1/2 -> Terminator1/1
  Demux/2 -> Terminator/1
  Switch/1 -> y/1
  computed torque switch/1 -> Switch/2
  MATLAB Function/1(tau) -> Switch/1
  end-effector attach/1 -> MATLAB Function/2(ee_att)
